simulink model "two_tank_model"  (Simulink 8.4)
settings: Solver=ode45  SolverMode=SingleTasking  StartTime=0.0  StopTime=1000  RelTol=1e-3
values from neighbouring files (symbols this model uses):
  A = 1.54    [two_tank_params.m]
  c_M = 12.0    (= 12)    [two_tank_params.m]
  h_max = 0.6    [two_tank_params.m]
  leakage = 0    [two_tank_params.m]
  q_bar_P = 1.5e-4    (= 0.00015)    [two_tank_params.m]
  u_nom = 1    [two_tank_params.m]
settings Model: Creator=Алексей  LastModifiedBy=Алексей  CovMetricSettings=dwe  CovHtmlReporting=off  covSaveCumulativeToWorkspaceVar=off  CovSaveSingleToWorkspaceVar=off  CovExternalEMLEnable=on  CovSFcnEnable=on
settings DataIOCC: LimitDataPoints=off  SaveFormat=StructureWithTime  SignalLoggingSaveFormat=Dataset  ReturnWorkspaceOutputs=on
settings OptimizationCC: ExpressionDepthLimit=128
settings DebuggingCC: UnderspecifiedInitializationDetection=Simplified  MergeDetectMultiDrivingBlocksExec=error  SolverPrmCheckMsg=none  FcnCallInpInsideContextMsg=EnableAllAsError  FrameProcessingCompatibilityMsg=error  StateNameClashWarn=none  SFUnexpectedBacktrackingDiag=error  SFNoUnconditionalDefaultTransitionDiag=error
settings HardwareCC: ProdBitPerPointer=64  ProdLargestAtomicFloat=Float  ProdIntDivRoundTo=Zero  ProdEndianess=LittleEndian  ProdHWDeviceType=Specified
settings ModelReferenceCC: PropagateSignalLabelsOutOfModel=on
settings SFSimCC: SimUseLocalCustomCode=on
settings RTWCC: RTWUseLocalCustomCode=on
settings GRTTargetCC: TargetLangStandard=C99 (ISO)  CombineOutputUpdateFcns=on  GRTInterface=off

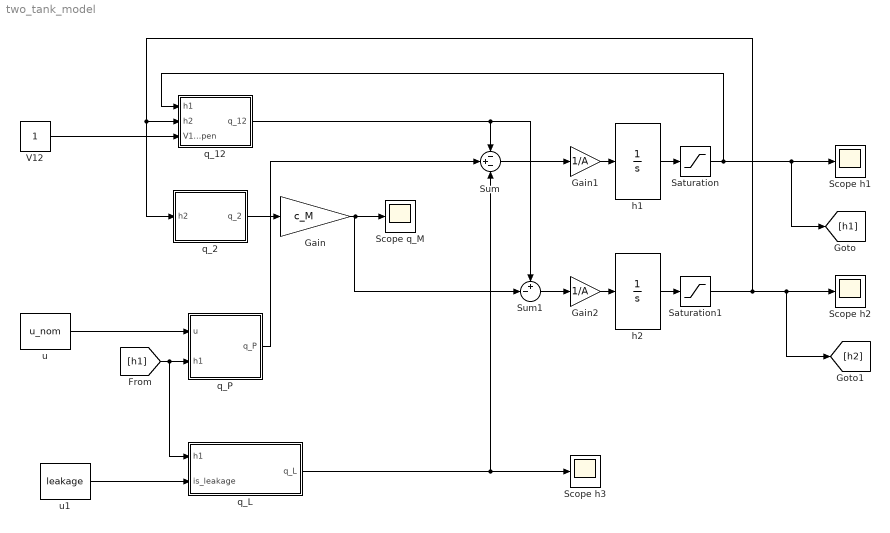
== system two_tank_model ==
  Gain : Gain  Gain=c_M
  Gain1 : Gain  Gain=1/A
  Gain2 : Gain  Gain=1/A
  Saturation : Saturate  UpperLimit=h_max  LowerLimit=0
  Saturation1 : Saturate  UpperLimit=h_max  LowerLimit=0
  Scope h1 : Scope
      settings: TimeRange=auto  MaxDataPoints=5000  SaveToWorkspace=off  SaveName=ScopeData  YMin=0.23308  YMax=0.32039  SampleTime=-1
  Scope h2 : Scope
      settings: TimeRange=auto  MaxDataPoints=5000  SaveToWorkspace=off  YMin=-0.01741  YMax=0.33527  SampleTime=-1
  Scope h3 : Scope
      settings: TimeRange=auto  MaxDataPoints=5000  SaveToWorkspace=off  SaveName=ScopeData3  YMin=-1.00000  YMax=1.00000  SampleTime=-1
  Scope q_M : Scope
      settings: TimeRange=auto  MaxDataPoints=5000  SaveToWorkspace=off  SaveName=ScopeData2  YMin=0.0002  YMax=0.00144  SampleTime=-1
  Sum : Sum  Inputs=-+-
  Sum1 : Sum  Inputs=+-|
  V12 : Constant
  h1 : Integrator  InitialCondition=0.3
  h2 : Integrator  InitialCondition=0.3
  q_12 : MATLAB Function  TreatAsAtomicUnit=on
      settings: PermitHierarchicalResolution=ParametersOnly
  q_2 : MATLAB Function  TreatAsAtomicUnit=on
      settings: PermitHierarchicalResolution=ParametersOnly
  q_L : MATLAB Function  TreatAsAtomicUnit=on
      settings: PermitHierarchicalResolution=ParametersOnly
  q_P : MATLAB Function  TreatAsAtomicUnit=on
      settings: PermitHierarchicalResolution=ParametersOnly
  u : Constant  Value=u_nom
  u1 : Constant  Value=leakage
  wires:
  V12/1 -> q_12/3(V12_is_open)
  h2/1 -> Saturation1/1
  q_12/1(q_12) -> Sum1/1, Sum/1
  q_2/1(q_2) -> Gain/1
  Gain/1 -> Sum1/2, Scope q_M/1
  [h1] -> q_L/1(h1), q_P/2(h1)
  u/1 -> q_P/1(u)
  u1/1 -> q_L/2(is_leakage)
  q_P/1(q_P) -> Sum/2
  q_L/1(q_L) -> Scope h3/1, Sum/3
  Sum/1 -> Gain1/1
  Gain1/1 -> h1/1
  Sum1/1 -> Gain2/1
  Gain2/1 -> h2/1
  h1/1 -> Saturation/1
  Saturation/1 -> q_12/1(h1), [h1], Scope h1/1
  Saturation1/1 -> [h2], Scope h2/1, q_2/1(h2), q_12/2(h2)

== matlab function q_2 ==
  data: h2 input double; q_2 output double; c_2 parameter double
function q_2 = fcn(h2, c_2)
if h2<=0
    q_2 = 0;
else
    q_2 = c_2 * sqrt(h2);
end

== matlab function q_12 ==
  data: h1 input double; q_12 output double; h2 input double; V12_is_open input double; c_12 parameter double
function q_12 = fcn(h1, h2, V12_is_open, c_12)
if V12_is_open == 0
    q_12 = 0;
else
    q_12 = c_12 * sign(h1 - h2) * sqrt(abs(h1 - h2));
end

== matlab function q_P ==
  data: u input double; q_P output double; h1 input double; h_max parameter double; q_bar_P parameter double
function q_P = fcn(u, h1, h_max, q_bar_P)
if h1 <= h_max
    q_P = u * q_bar_P;
else
    q_P = 0;
end

== matlab function q_L ==
  data: h1 input double; q_L output double; is_leakage input double; c_L parameter double
function q_L = fcn(h1, is_leakage, c_L)
if h1 > 0 && is_leakage ~= 0
    q_L = c_L * sqrt(h1);
else
    q_L = 0;
end
